simulink model "Final_Model"  (R2020a)
settings: Solver=VariableStepAuto  StartTime=0.0  StopTime=15  RelTol=1e-3
model workspace (MAT data in the model file):
  breaker_state : Simulink.Parameter (value not decoded)
  cap_state : Simulink.Parameter (value not decoded)
symbols that are objects in the model workspace (value not decoded): breaker_state
undefined symbols (not defined in the file or in its folder): state
libraries: ee_lib x78, nesl_utility x49, fl_lib x10, simulink x2
(part 2 of 2)

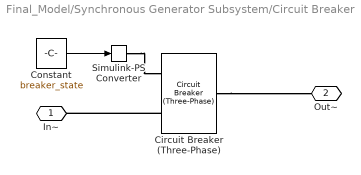
== system Final_Model/Synchronous Generator Subsystem/Circuit Breaker ==
  Circuit Breaker (Three-Phase) : ee_lib/Switches & Breakers/Circuit Breaker (Three-Phase)  R_closed=0.001 Ohm  G_open=1e-6 1/Ohm  threshold=0.5 V
      settings: SourceProductBaseCode=PS  InternalSimscapePortConfiguration="{\"Bottom\":[],\"Left\":[{\"id\":\"vT\",\"label\":\"vT\",\"type\":\"input\"},{\"id\":\"N1\",\"label\":\"~1\",\"type\":\"foundation.electrical.three_phase\"}],\"Right\":[{\"id\":\"N2\",\"label\":\"~2\",\"type\":\"foundation.electrical.three_phase\"}],\"Top\":[]}"
  Constant : Constant  Value=breaker_state
  Simulink-PS Converter : nesl_utility/Simulink-PS Converter  PhysicalDomain=network_engine_domain  SubClassName=ps_input  LeftPortType=input  RightPortType=output  PseudoPeriodic=off  Frequencies=[]  NoiseDistribution=none  NoiseParameters=[]  Unit=1  AffineConversion=off  FilteringAndDerivatives=provide  SimscapeFilterOrder=1  InputFilterTimeConstant=0.001  UdotUserProvided=0
  In~ : PMIOPort  Side=Left
  Out~ : PMIOPort  Port=2  Side=Right
  wires:
  Constant/1 -> Simulink-PS Converter/1
  connections:
  Simulink-PS Converter/RConn1 -- Circuit Breaker (Three-Phase)/LConn1
  Circuit Breaker (Three-Phase)/LConn2 -- In~/RConn1
  Circuit Breaker (Three-Phase)/RConn1 -- Out~/RConn1

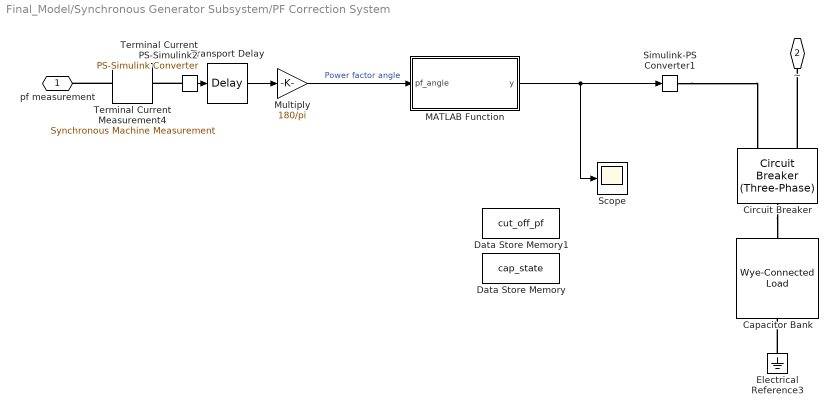
== system Final_Model/Synchronous Generator Subsystem/PF Correction System ==
  Capacitor Bank : ee_lib/Passive/RLC Assemblies/Wye-Connected Load  parameterization=2  component_structure=1  component_structure_PQ=3  R=1 Ohm  L=0.001 H  C=1e-6 F  IL0=[ 0 0 0 ] A  VC0=[ 0 0 0 ] V  R_parasitic=1e-6 Ohm  G_parasitic=1e-6 1/Ohm  VRated=24e3 V  FRated=60 Hz  P=1500e6 W  Qpos=1000e6 V*A  Qneg=cap_reactive_power V*A  Vmag0=0 V  Vang0=0 deg  Freq0=60 Hz  R_parasitic_PQ=1e-6 Ohm  G_parasitic_PQ=1e-6 1/Ohm
      settings: SourceProductBaseCode=PS
  Circuit Breaker : ee_lib/Switches & Breakers/Circuit Breaker (Three-Phase)  R_closed=0.001 Ohm  G_open=1e-4 1/Ohm  threshold=0.5 V
      settings: SourceProductBaseCode=PS  InternalSimscapePortConfiguration="{\"Bottom\":[],\"Left\":[{\"id\":\"vT\",\"label\":\"vT\",\"type\":\"input\"},{\"id\":\"N1\",\"label\":\"~1\",\"type\":\"foundation.electrical.three_phase\"}],\"Right\":[{\"id\":\"N2\",\"label\":\"~2\",\"type\":\"foundation.electrical.three_phase\"}],\"Top\":[]}"
  Data Store Memory : DataStoreMemory  DataStoreName=cap_state  InitialValue=1  ShowAdditionalParam=off  OutDataTypeStr=double
  Data Store Memory1 : DataStoreMemory  DataStoreName=cut_off_pf  InitialValue=0.9  ShowAdditionalParam=off  OutDataTypeStr=double
  Electrical Reference3 : fl_lib/Electrical/Electrical Elements/Electrical Reference
      settings: SourceProductBaseCode=MT,SS
  MATLAB Function : MATLAB Function  TreatAsAtomicUnit=on
  Multiply : Gain  Gain=180/pi
  Scope : Scope
  Simulink-PS Converter1 : nesl_utility/Simulink-PS Converter  PhysicalDomain=network_engine_domain  SubClassName=ps_input  LeftPortType=input  RightPortType=output  PseudoPeriodic=off  Frequencies=[]  NoiseDistribution=none  NoiseParameters=[]  Unit=1  AffineConversion=off  FilteringAndDerivatives=zero  SimscapeFilterOrder=1  InputFilterTimeConstant=0.001  UdotUserProvided=1
      settings: SourceProductBaseCode=MT,SS
  Terminal Current Measurement4 : ee_lib/Electromechanical/Synchronous/Synchronous Machine Measurement  output_idx=16
      settings: SourceProductBaseCode=PS  InternalSimscapePortConfiguration="{\"Bottom\":[],\"Left\":[{\"id\":\"pu_input\",\"label\":\"pu\",\"type\":\"input\"}],\"Right\":[{\"id\":\"pu_output\",\"label\":\"o\",\"type\":\"output\"}],\"Top\":[]}"
  Terminal Current PS-Simulink2 : nesl_utility/PS-Simulink Converter  PhysicalDomain=network_engine_domain  SubClassName=ps_output  LeftPortType=input  RightPortType=output  PseudoPeriodic=off  Frequencies=[]  Unit=1  AffineConversion=off
      settings: SourceProductBaseCode=MT,SS
  Transport Delay : TransportDelay  DelayTime=transport_delay
  pf measurement : PMIOPort  Side=Left
  ~ : PMIOPort  Port=2  Side=Left
  wires:
  Terminal Current PS-Simulink2/1 -> Transport Delay/1
  Multiply/1 -> MATLAB Function/1(pf_angle)  "Power factor angle"
  Transport Delay/1 -> Multiply/1
  MATLAB Function/1(y) -> Scope/1, Simulink-PS Converter1/1
  connections:
  Circuit Breaker/RConn1 -- Capacitor Bank/LConn1
  Terminal Current Measurement4/LConn1 -- pf measurement/RConn1
  Simulink-PS Converter1/RConn1 -- Circuit Breaker/LConn1
  Terminal Current PS-Simulink2/LConn1 -- Terminal Current Measurement4/RConn1
  Electrical Reference3/LConn1 -- Capacitor Bank/RConn1
  Circuit Breaker/LConn2 -- ~/RConn1

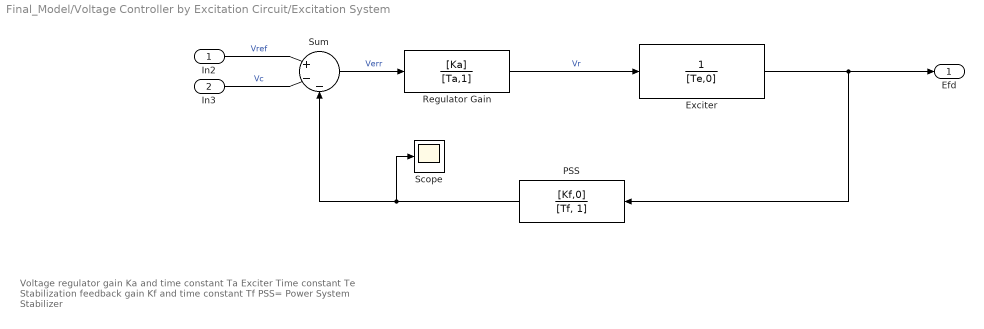
== system Final_Model/Voltage Controller by Excitation Circuit/Excitation System ==
  note: Voltage regulator gain Ka and time constant Ta
      | Exciter Time constant Te
      | Stabilization feedback gain Kf and time constant Tf
      | PSS= Power System Stabilizer
  In2 : Inport
  In3 : Inport  Port=2
  Exciter : TransferFcn  Denominator=[Te,0]
  PSS : TransferFcn  Numerator=[Kf,0]  Denominator=[Tf, 1]
  Regulator Gain : TransferFcn  Numerator=[Ka]  Denominator=[Ta,1]
  Scope : Scope
  Sum : Sum  Inputs=|+--
  Efd : Outport
  wires:
  Regulator Gain/1 -> Exciter/1  "Vr"
  Sum/1 -> Regulator Gain/1  "Verr"
  In3/1 -> Sum/2  "Vc"
  In2/1 -> Sum/1  "Vref"
  PSS/1 -> Scope/1, Sum/3
  Exciter/1 -> PSS/1, Efd/1

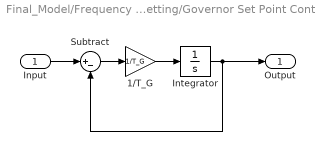
== system Final_Model/Frequency Controller by Governor set point setting/Governor Set Point Controller/1st order Governor Response ==
  Input : Inport
  1/T_G : Gain  Gain=1/T_G
  Integrator : Integrator  InitialCondition=pu_torque0
  Subtract : Sum  Inputs=|+-
  Output : Outport
  wires:
  Subtract/1 -> 1/T_G/1
  Integrator/1 -> Output/1, Subtract/2
  Input/1 -> Subtract/1
  1/T_G/1 -> Integrator/1

== system Final_Model/Frequency Controller by Governor set point setting/Governor Set Point Controller/Governor Set point Controller ==
  Reference Speed : Inport
  pu_rotor_speed : Inport  Port=2
  PID Controller : simulink/Continuous/PID Controller  Controller=PID  Form=Parallel  TimeDomain=Discrete-time  UseExternalTs=off  SampleTime=-1  IntegratorMethod=Forward Euler  FilterMethod=Forward Euler  ControllerParametersSource=internal  P=-13.7673478847226  I=-18.789489771293  D=-2.5218868379945  UseFilter=off  N=294.375672178551  TunerSelectOption=Transfer Function Based (PID Tuner App)  InitialConditionSource=internal  InitialConditionForIntegrator=0  InitialConditionForFilter=0  DifferentiatorICPrevScaledInput=0  ExternalReset=none  TrackingMode=off  Kt=1  LimitOutput=off  UpperSaturationLimit=inf  LowerSaturationLimit=-inf  LinearizeAsGain=on  AntiWindupMode=none  Kb=1  POutMin=[]  POutMax=[]  IOutMin=[]  IOutMax=[]  DOutMin=[]  DOutMax=[]  NOutMin=[]  NOutMax=[]  SumOutMin=[]  SumOutMax=[]  SaturationOutMin=[]  SaturationOutMax=[]  PParamMin=[]  PParamMax=[]  IParamMin=[]  IParamMax=[]  DParamMin=[]  DParamMax=[]  NParamMin=[]  NParamMax=[]  KbParamMin=[]  KbParamMax=[]  KtParamMin=[]  KtParamMax=[]  KbOutMin=[]  KbOutMax=[]  KtOutMin=[]  KtOutMax=[]  IntegratorOutMin=[]  IntegratorOutMax=[]  FilterOutMin=[]  FilterOutMax=[]  SumI1OutMin=[]  SumI1OutMax=[]  SumI2OutMin=[]  SumI2OutMax=[]  SumI3OutMin=[]  SumI3OutMax=[]  SumI4OutMin=[]  SumI4OutMax=[]  SumDOutMin=[]  SumDOutMax=[]  DifferentiatorOutMin=[]  DifferentiatorOutMax=[]  FilterDiffOutCoefMin=[]  FilterDiffOutCoefMax=[]  ReciprocalOutMin=[]  ReciprocalOutMax=[]  SumDenOutMin=[]  SumDenOutMax=[]  SumNumOutMin=[]  SumNumOutMax=[]  DivideOutMin=[]  DivideOutMax=[]  UdiffTsProdOutMin=[]  UdiffTsProdOutMax=[]  NTsProdOutMin=[]  NTsProdOutMax=[]  UintegralTsProdOutMin=[]  UintegralTsProdOutMax=[]  UngainTsProdOutMin=[]  UngainTsProdOutMax=[]  IntegratorContinuousStateAttributes=''  IntegratorStateMustResolveToSignalObject=off  IntegratorRTWStateStorageClass=Auto  FilterContinuousStateAttributes=''  FilterStateMustResolveToSignalObject=off  FilterRTWStateStorageClass=Auto  ParallelPVariant=InternalParameters  IdealPVariant=Disabled  IVariant=InternalParameters  DVariant=InternalParameters  IntegratorVariant=Discrete  SatVariant=Disabled  AWVariant=Passthrough  PCopyVariant=Disabled  TRVariant=Disabled  FdbkBlocksVariant=Forward  IdealPFdbkVariant=Disabled  SatFdbkVariant=Disabled  DerivativeFilterVariant=Differentiator  NVariant=Passthrough  NCopyVariant=Disabled_SignalSpec  FilterICVariant=InternalICsDifferentiator  IntegratorICVariant=InternalICs  ExternalResetVariant=Disabled  TRSumVariant=Passthrough  SumFdbkVariant=Disabled  SumVariant=Sum_PID  TsampFilterVariant=InternalTs  TsampNgainVariant=Passthrough  TsampIntegralVariant=Passthrough
  Sum : Sum  Inputs=|+-
  Governor Set Point : Outport
  wires:
  Sum/1 -> PID Controller/1  "Error signal"
  PID Controller/1 -> Governor Set Point/1  "Governor Set Point"
  pu_rotor_speed/1 -> Sum/1
  Reference Speed/1 -> Sum/2

== matlab function Final_Model/Synchronous Generator Subsystem/PF Correction System/MATLAB Function ==
  settings: updateMethod=DISCRETE
  data: pf_angle input; y output; cap_state data_store_memory; cut_off_pf data_store_memory
function y = fcn(pf_angle)


global cap_state;
global cut_off_pf;

cut_off_angle = acos(0.9)*180/pi;

if(cap_state == 1)
    if(pf_angle > cut_off_angle)
        cap_state = 0;
    end
else
    if(pf_angle < 0)
        cap_state = 1;
    end
end
    
y = cap_state;
